simulink model "hardwar_harness"  (R2021a)
settings: Solver=FixedStepAuto  StartTime=0.0  StopTime=inf  RelTol=1e-3
libraries: arduinolib x8, arduinosensorlib x1
settings Model: SILPILModeSetting=veronly  ExtModeTrigDuration=2  Creator=Nabil  LastModifiedBy=Nabil
settings OptimizationCC: EnhancedBackFolding=on  PassReuseOutputArgsAs=Individual arguments  ZeroExternalMemoryAtStartup=off  ZeroInternalMemoryAtStartup=off  MaxStackSize=64  OptimizeBlockOrder=speed  DifferentSizesBufferReuse=on  OptimizationCustomize=off  EfficientTunableParamExpr=on
settings DebuggingCC: ParameterTunabilityLossMsg=error
settings HardwareCC: ProdBitPerInt=16  ProdBitPerPointer=16  ProdBitPerSizeT=16  ProdBitPerPtrDiffT=16  ProdLargestAtomicFloat=None  ProdWordSize=8  ProdHWDeviceType=Atmel->AVR
settings SFSimCC: MATLABDynamicMemAlloc=off
settings RTWCC: SystemTargetFile=ert.tlc  HardwareBoard=Arduino Uno  TemplateMakefile=ert_default_tmf  Toolchain=Arduino AVR
settings CodeAppCC: ForceParamTrailComments=on  IgnoreCustomStorageClasses=off  OperatorAnnotations=on  SimulinkDataObjDesc=on  SFDataObjDesc=on  InsertBlockDesc=on
settings ERTTargetCC: SupportContinuousTime=on  SupportVariableSizeSignals=on  ExtModeStaticAllocSize=250

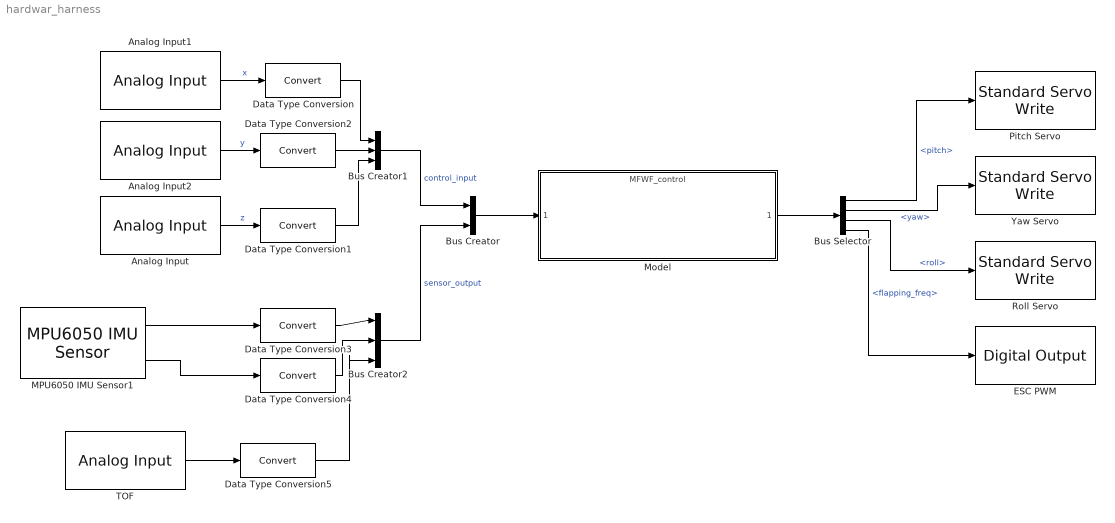
== system hardwar_harness ==
  Analog Input : arduinolib/Analog Input  pinNumber=3  ReadResultsOnly=off  ConversionTriggerSource=Software  ExternalTriggerType=uint32( 0 )  OutputDataType=uint16  EnableConversionCompleteNotify=off  EnableOuputStatus=off  SampleTime=-1  blockPlatform=arduino
  Analog Input1 : arduinolib/Analog Input  pinNumber=1  ReadResultsOnly=off  ConversionTriggerSource=Software  ExternalTriggerType=uint32( 0 )  OutputDataType=uint16  EnableConversionCompleteNotify=off  EnableOuputStatus=off  SampleTime=-1  blockPlatform=arduino
  Analog Input2 : arduinolib/Analog Input  pinNumber=2  ReadResultsOnly=off  ConversionTriggerSource=Software  ExternalTriggerType=uint32( 0 )  OutputDataType=uint16  EnableConversionCompleteNotify=off  EnableOuputStatus=off  SampleTime=-1  blockPlatform=arduino
  Bus Creator : BusCreator  Inputs=2
  Bus Creator1 : BusCreator  Inputs=3
  Bus Creator2 : BusCreator  Inputs=3
  Bus Selector : BusSelector  OutputSignals=pitch,yaw,roll,flapping_freq
  Data Type Conversion{,1..5} (6 alike) : DataTypeConversion
  ESC PWM : arduinolib/Digital Output  pinNumber=10  Direction=output  blockPlatform=arduino
  MPU6050 IMU Sensor1 : arduinosensorlib/MPU6050 IMU Sensor  SlaveAddress=0x68  Accel=on  AngularRate=on  Temperature=off  Status=off  EulerAngles=off  Quat=off  AccelRange=2G  GyroRange=250 dps  DmpOdr=200 Hz  Dlpf=Accelerometer: 184Hz, Gyroscope: 188Hz  SampleTime=-1
      settings: SourceProductBaseCode=ARDUINO
  Model : ModelReference  ModelNameDialog=MFWF_control.slx  SimulationMode=Normal  ModelReferenceVersion=8.14
  Pitch Servo : arduinolib/Standard Servo Write  pinNumber=9  ServoIndex=0  blockPlatform=ARDUINO
  Roll Servo : arduinolib/Standard Servo Write  pinNumber=7  ServoIndex=0  blockPlatform=ARDUINO
  TOF : arduinolib/Analog Input  pinNumber=4  ReadResultsOnly=off  ConversionTriggerSource=Software  ExternalTriggerType=uint32( 0 )  OutputDataType=uint16  EnableConversionCompleteNotify=off  EnableOuputStatus=off  SampleTime=-1  blockPlatform=arduino
  Yaw Servo : arduinolib/Standard Servo Write  pinNumber=8  ServoIndex=0  blockPlatform=ARDUINO
  wires:
  Model/1 -> Bus Selector/1
  Bus Selector/3 -> Roll Servo/1  "<roll>"
  Bus Selector/4 -> ESC PWM/1  "<flapping_freq>"
  Bus Selector/1 -> Pitch Servo/1  "<pitch>"
  Bus Selector/2 -> Yaw Servo/1  "<yaw>"
  MPU6050 IMU Sensor1/1 -> Data Type Conversion3/1
  Analog Input1/1 -> Data Type Conversion/1  "x"
  Analog Input/1 -> Data Type Conversion1/1  "z"
  Bus Creator1/1 -> Bus Creator/1  "control_input"
  MPU6050 IMU Sensor1/2 -> Data Type Conversion4/1
  TOF/1 -> Data Type Conversion5/1
  Bus Creator2/1 -> Bus Creator/2  "sensor_output"
  Bus Creator/1 -> Model/1
  Data Type Conversion/1 -> Bus Creator1/1
  Data Type Conversion1/1 -> Bus Creator1/3
  Data Type Conversion2/1 -> Bus Creator1/2
  Analog Input2/1 -> Data Type Conversion2/1  "y"
  Data Type Conversion3/1 -> Bus Creator2/1
  Data Type Conversion4/1 -> Bus Creator2/2
  Data Type Conversion5/1 -> Bus Creator2/3
